simulink model "audio_band_adc_"  (Simulink 10.3)
settings: Solver=FixedStepDiscrete  StartTime=0.0  StopTime=1  RelTol=1e-3  EnableMultiTasking=on
undefined symbols (not defined in the file): c, dfilt, Fs, modctrl
libraries: dspsrcs4 x2, dspobslib x1
settings Model: Creator=amyles  LastModifiedBy=samir
settings DataIOCC: MaxDataPoints=50000  SignalLoggingSaveFormat=Dataset
settings OptimizationCC: DefaultParameterBehavior=Inlined
settings DebuggingCC: SolverPrmCheckMsg=warning
settings ModelReferenceCC: ModelReferenceNumInstancesAllowed=Single

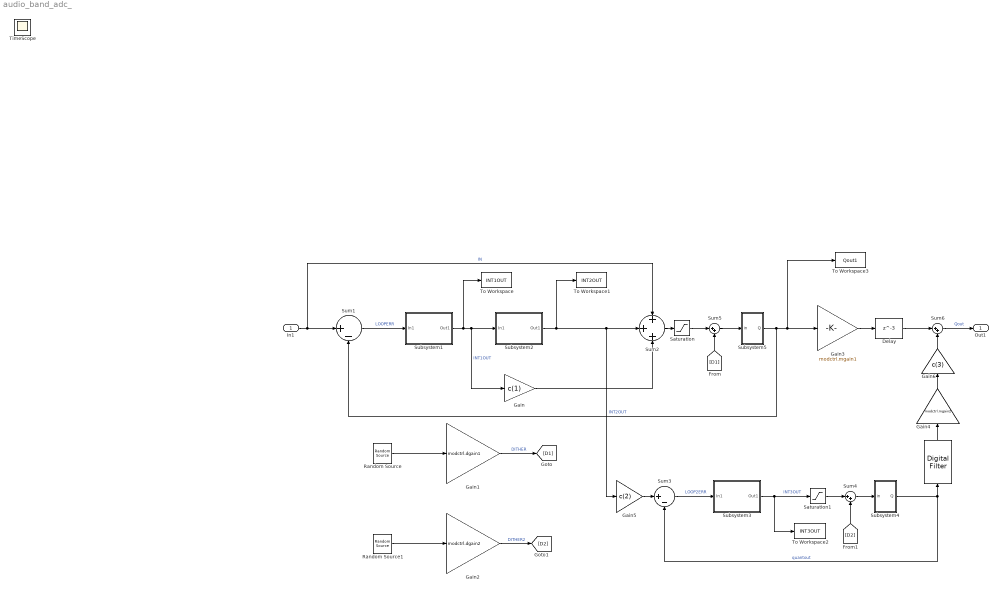
== system audio_band_adc_ ==
  In1 : Inport
  " " : dspobslib/Digital Filter  TypePopup=FIR (all zeros)  IIRFiltStruct=Direct form II transposed  AllPoleFiltStruct=Direct form  FIRFiltStruct=Direct form  CoeffSource=Specify via dialog  NumCoeffs=[1 -2 1]  DenCoeffs=[1 0.1]  BiQuadCoeffs=[1 0.3 0.4 1 0.1 0.2]  LatticeCoeffs=[0.2 0.4]  denIgnore=on  FiltPerSampPopup=One filter per frame  IC=0  ICnum=0  ICden=0  roundingMode=Floor  overflowMode=off  ScaleValues=1  scaleValueFracLength=14  stageInFracLength=15  stageOutFracLength=15  FilterSource=Specify via dialog  dfiltObjectName=dfilt.dffir([1 2 1])  InputProcessing=Inherited (this choice will be removed - see release notes)
      settings: AttributesFormatString=NTF1 = (1-z^-1)^2  SourceProductBaseCode=DS
  Delay : Delay  DelayLength=3  InitialCondition=0
  Gain : Gain  Gain=c(1)
  Gain1 : Gain  Gain=modctrl.dgain1
      settings: AttributesFormatString=Dither level adjust
  Gain2 : Gain  Gain=modctrl.dgain2
      settings: AttributesFormatString=Dither level adjust
  Gain3 : Gain  Gain=modctrl.mgain1
  Gain4 : Gain  Gain=modctrl.mgain2
  Gain5 : Gain  Gain=c(2)
      settings: AttributesFormatString=Option to scale input\nfor saturation control...
  Gain6 : Gain  Gain=c(3)
      settings: AttributesFormatString=Option to un-scale input\npost saturation control...
  Random Source : dspsrcs4/Random Source  SrcType=Uniform  NormMethod=Ziggurat  CltLength=12  MinVal=-1  MaxVal=1  MeanVal=0  VarVal=1  RepMode=Not repeatable  rawSeed=1  IsInherit=off  SampMode=Discrete  SampTime=1/Fs  SampFrame=1  DataType=Double  OutComplex=Real  OutputFrames=on
      settings: AttributesFormatString=Dither source
  Random Source1 : dspsrcs4/Random Source  SrcType=Uniform  NormMethod=Ziggurat  CltLength=12  MinVal=-1  MaxVal=1  MeanVal=0  VarVal=1  RepMode=Not repeatable  rawSeed=1  IsInherit=off  SampMode=Discrete  SampTime=1/Fs  SampFrame=1  DataType=Double  OutComplex=Real  OutputFrames=on
      settings: AttributesFormatString=Dither source
  Saturation : Saturate  UpperLimit=modctrl.qsatin1  LowerLimit=-(modctrl.qsatin1)
  Saturation1 : Saturate  UpperLimit=modctrl.qsatin2  LowerLimit=-(modctrl.qsatin2)
  Subsystem1 : Subsystem
      settings: AttributesFormatString=Leaky delaying int
  Subsystem2 : Subsystem
      settings: AttributesFormatString=Leaky delaying int
  Subsystem3 : Subsystem
      settings: AttributesFormatString=Leaky delaying int
  Subsystem4 : Subsystem
      settings: AttributesFormatString=3-bit quantiser
  Subsystem5 : Subsystem
      settings: AttributesFormatString=3-bit quantiser
  Sum1 : Sum  Inputs=|+-
      settings: AttributesFormatString=Modulator input\nloop servo error (input - fbk)
  Sum2 : Sum  Inputs=+++
  Sum3 : Sum  Inputs=|+-
      settings: AttributesFormatString=Modulator input\nloop servo error (input - fbk)
  Sum4 : Sum  Inputs=|++
  Sum5 : Sum  Inputs=|++
  Sum6 : Sum  Inputs=|++
  To Workspace : ToWorkspace  VariableName=INT1OUT  SampleTime=-1
  To Workspace1 : ToWorkspace  VariableName=INT2OUT  SampleTime=-1
  To Workspace2 : ToWorkspace  VariableName=INT3OUT  SampleTime=-1
  To Workspace3 : ToWorkspace  VariableName=Qout1  SampleTime=-1
  Out1 : Outport
  TimeScope : Scope
  wires:
  " "/1 -> Gain4/1
  [D2] -> Sum4/2
  Subsystem2/1(Out1) -> Sum2/2, Gain5/1, To Workspace1/1  "INT2OUT"
  Sum4/1 -> Subsystem4/1(in)
  Gain3/1 -> Delay/1
  Sum6/1 -> Out1/1  "Qout"
  Gain2/1 -> [D2]  "DITHER2"
  Subsystem5/1(Q) -> Sum1/2, To Workspace3/1, Gain3/1
  Gain5/1 -> Sum3/1
  Sum5/1 -> Subsystem5/1(in)
  Saturation1/1 -> Sum4/1
  Random Source1/1 -> Gain2/1
  Subsystem3/1(Out1) -> Saturation1/1, To Workspace2/1  "INT3OUT"
  Sum3/1 -> Subsystem3/1(In1)  "LOOP2ERR"
  Sum2/1 -> Saturation/1
  Gain/1 -> Sum2/3
  Subsystem1/1(Out1) -> Subsystem2/1(In1), Gain/1, To Workspace/1  "INT1OUT"
  [D1] -> Sum5/2
  In1/1 -> Sum1/1, Sum2/1  "IN"
  Delay/1 -> Sum6/1
  Gain6/1 -> Sum6/2
  Gain4/1 -> Gain6/1
  Gain1/1 -> [D1]  "DITHER"
  Saturation/1 -> Sum5/1
  Sum1/1 -> Subsystem1/1(In1)  "LOOPERR"
  Subsystem4/1(Q) -> Sum3/2, " "/1  "quantout"
  Random Source/1 -> Gain1/1

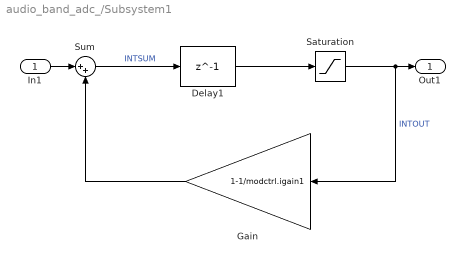
== system audio_band_adc_/Subsystem1 ==
  In1 : Inport
  Delay1 : Delay  DelayLength=1  InitialCondition=0
  Gain : Gain  Gain=1-1/modctrl.igain1
      settings: AttributesFormatString=Integrator leakage
  Saturation : Saturate  UpperLimit=modctrl.isat1  LowerLimit=-(modctrl.isat1)
  Sum : Sum  Inputs=|++
      settings: AttributesFormatString=Integrator summer
  Out1 : Outport
  wires:
  Sum/1 -> Delay1/1  "INTSUM"
  Gain/1 -> Sum/2
  Saturation/1 -> Gain/1, Out1/1  "INTOUT"
  Delay1/1 -> Saturation/1
  In1/1 -> Sum/1

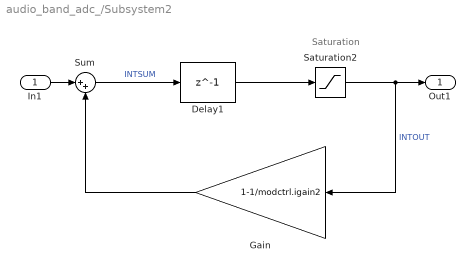
== system audio_band_adc_/Subsystem2 ==
  note: Saturation
  In1 : Inport
  Delay1 : Delay  DelayLength=1  InitialCondition=0
  Gain : Gain  Gain=1-1/modctrl.igain2
      settings: AttributesFormatString=Integrator leakage
  Saturation2 : Saturate  UpperLimit=modctrl.isat2  LowerLimit=-(modctrl.isat2)
  Sum : Sum  Inputs=|++
      settings: AttributesFormatString=Integrator summer
  Out1 : Outport
  wires:
  In1/1 -> Sum/1
  Delay1/1 -> Saturation2/1
  Saturation2/1 -> Out1/1, Gain/1  "INTOUT"
  Gain/1 -> Sum/2
  Sum/1 -> Delay1/1  "INTSUM"

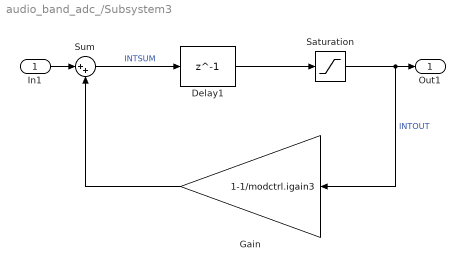
== system audio_band_adc_/Subsystem3 ==
  In1 : Inport
  Delay1 : Delay  DelayLength=1  InitialCondition=0
  Gain : Gain  Gain=1-1/modctrl.igain3
      settings: AttributesFormatString=Integrator leakage
  Saturation : Saturate  UpperLimit=modctrl.isat3  LowerLimit=-(modctrl.isat3)
  Sum : Sum  Inputs=|++
      settings: AttributesFormatString=Integrator summer
  Out1 : Outport
  wires:
  In1/1 -> Sum/1
  Delay1/1 -> Saturation/1
  Saturation/1 -> Out1/1, Gain/1  "INTOUT"
  Gain/1 -> Sum/2
  Sum/1 -> Delay1/1  "INTSUM"

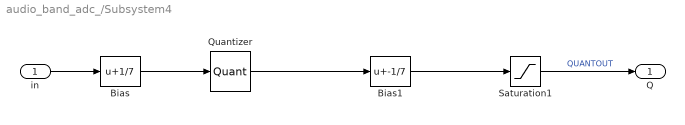
== system audio_band_adc_/Subsystem4 ==
  in : Inport
  Bias : Bias  Bias=1/7
      settings: AttributesFormatString=Need offset to give\nMID-RISE quantiser
  Bias1 : Bias  Bias=-1/7
  Quantizer : Quantizer  QuantizationInterval=2/7  LinearizeAsGain=off
  Saturation1 : Saturate  UpperLimit=1  LowerLimit=-1
      settings: AttributesFormatString=Limit quantiser\noutput to +/-1
  Q : Outport
  wires:
  Bias/1 -> Quantizer/1
  Quantizer/1 -> Bias1/1
  Bias1/1 -> Saturation1/1
  in/1 -> Bias/1
  Saturation1/1 -> Q/1  "QUANTOUT"

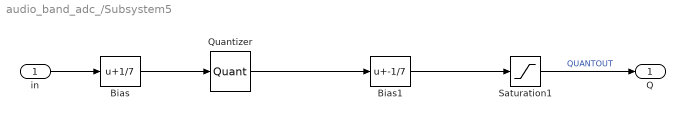
== system audio_band_adc_/Subsystem5 ==
  in : Inport
  Bias : Bias  Bias=1/7
      settings: AttributesFormatString=Need offset to give\nMID-RISE quantiser
  Bias1 : Bias  Bias=-1/7
  Quantizer : Quantizer  QuantizationInterval=2/7  LinearizeAsGain=off
  Saturation1 : Saturate  UpperLimit=1  LowerLimit=-1
      settings: AttributesFormatString=Limit quantiser\noutput to +/-1
  Q : Outport
  wires:
  Bias/1 -> Quantizer/1
  Quantizer/1 -> Bias1/1
  Bias1/1 -> Saturation1/1
  in/1 -> Bias/1
  Saturation1/1 -> Q/1  "QUANTOUT"
